simulink model "ammclib_amclib_FW_speed_loop_s32k14x"  (Simulink 9.0)
settings: Solver=FixedStepDiscrete  StartTime=0.0  StopTime=10  FixedStep=0.001  RelTol=1e-3  EnableMultiTasking=on
InitFcn:
  | mbd_s32k_consistency_checks(bdroot(gcs));
undefined symbols (not defined in the file or in its folder): LQFP
libraries: ammclib_bam_s32k14x x8, simulink x4, mbd_s32k1xx_ec_toolbox x2
Description:
  | This model tests the AMMCLIB AMCLIB Field Weakening Speed Loop blocks
  | 
  | Validation:
  | - Run the model in Simulation and compare the Inputs vs Outputs results.
  | - Open Freemaster (ammclib_amclib_FW_speed_loop_s32k14x.pmp) and compare the HW results against the Simulated ones
settings Model: Creator=NXP MBDT Team  LastModifiedBy=nxf35172
settings DataIOCC: ExternalInput=off  InitialState=off  LimitDataPoints=on  SaveOutput=off  SignalLogging=off  SaveTime=off
settings OptimizationCC: DefaultParameterBehavior=Inlined  LifeSpan=1
settings DebuggingCC: SolverPrmCheckMsg=warning  InheritedTsInSrcMsg=none  SingleTaskRateTransMsg=error  ParameterPrecisionLossMsg=none  UnconnectedInputMsg=error  UnconnectedOutputMsg=error  UnconnectedLineMsg=error  AllowSymbolicDim=off  UnknownTsInhSupMsg=error  StateNameClashWarn=warning
settings HardwareCC: ProdLargestAtomicInteger=Long  ProdLargestAtomicFloat=Double  ProdEndianess=LittleEndian  ProdHWDeviceType=ARM Compatible->ARM Cortex
settings SFSimCC: MATLABDynamicMemAlloc=off
settings RTWCC: SystemTargetFile=mbd_s32k.tlc  MakeCommand=mbd_s32k_make_rtw COPY_MDLREF_INCLUDES=0  TemplateMakefile=mbd_s32k.tmf  Description=Model Based Design Toolbox S32K14x Code Generation Target
settings CodeAppCC: IgnoreCustomStorageClasses=off
settings STFCustomTargetCC: CombineOutputUpdateFcns=on  ERTCustomFileBanners=on  SupportContinuousTime=off  SupportNonInlinedSFcns=off  RemoveResetFunc=on  MATLABClassNameForMDSCustomization=Simulink.SoftwareTarget.ERTCustomization  GRTInterface=off  SystemTargetFile=mbd_s32k14.tlc
settings ERTTargetCC: MultiwordLength=2048  ParMdlRefBuildCompliant=off  CompOptLevelCompliant=off  ConcurrentExecutionCompliant=off  ModelStepFunctionPrototypeControlCompliant=off  CPPClassGenCompliant=off  UseToolchainInfoCompliant=off  InlinedParameterPlacement=NonHierarchical  ERTCustomFileTemplate=example_file_process.tlc  ConvertIfToSwitch=off  SuppressUnreachableDefaultCases=off

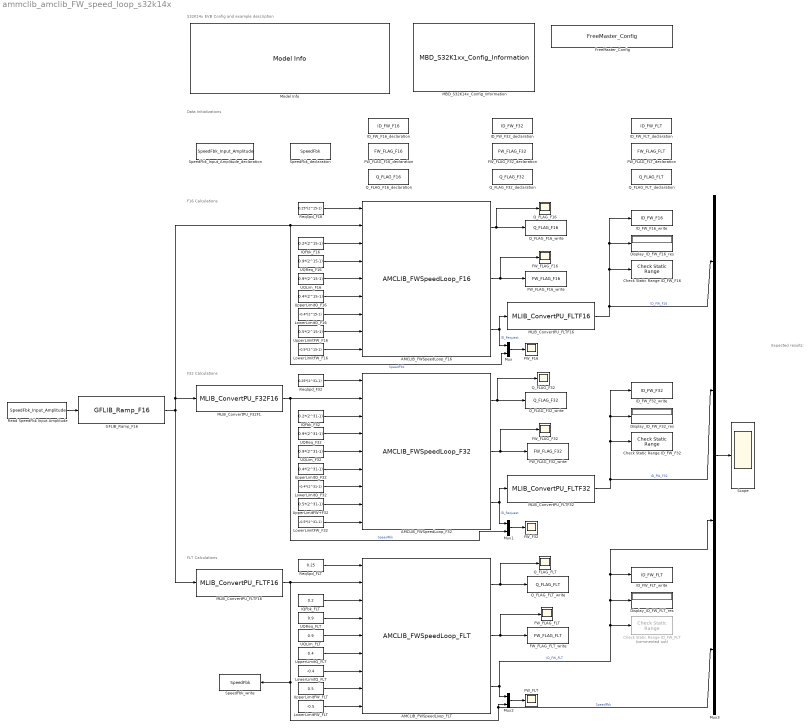
== system ammclib_amclib_FW_speed_loop_s32k14x ==
  note: Expected results:
  note: S32K14x EVB Config and example description
  note: Data Initializations
  note: F16 Calculations
  note: F32 Calculations
  note: FLT Calculations
  AMCLIB_FWSpeedLoop_F16 : ammclib_bam_s32k14x/AMCLIB/bam_f16/AMCLIB_FWSpeedLoop_F16  u16NSamplesW=3  u16NSamplesFW=3  f16PropGainQ=0.001*(2^15-1)  s16PropGainShiftQ=0  f16IntegGainQ=0.0005*(2^15-1)  s16IntegGainShiftQ=0  f16PropGainFW=0.02*(2^15-1)  s16PropGainShiftFW=0  f16IntegGainFW=0.002*(2^15-1)  s16IntegGainShiftFW=0  f32RampUp=0.001*(2^15-1)  f32RampDown=0.001*(2^15-1)
  AMCLIB_FWSpeedLoop_F32 : ammclib_bam_s32k14x/AMCLIB/bam_f32/AMCLIB_FWSpeedLoop_F32  u16NSamplesW=3  u16NSamplesFW=3  f32PropGainQ=0.001*(2^31-1)  s16PropGainShiftQ=0  f32IntegGainQ=0.0005*(2^31-1)  s16IntegGainShiftQ=0  f32PropGainFW=0.02*(2^31-1)  s16PropGainShiftFW=0  f32IntegGainFW=0.002*(2^31-1)  s16IntegGainShiftFW=0  f32RampUp=0.001*(2^31-1)  f32RampDown=0.001*(2^31-1)
  AMCLIB_FWSpeedLoop_FLT : ammclib_bam_s32k14x/AMCLIB/bam_flt/AMCLIB_FWSpeedLoop_FLT  fltLambdaW=0.5  fltLambdaFW=0.5  fltPropGainQ=0.001  fltIntegGainQ=0.0005  fltPropGainFW=0.02  fltIntegGainFW=0.002  fltRampUp=0.001  fltRampDown=0.001  fltUmaxDivImax=1
  "Check Static Range ID_FW_F16 " : simulink/Model Verification/Check  Static Range  Description=0 <= u <= 0.707*(2^15-1)  max=0.707*(2^15-1)  max_included=on  min=0  min_included=on  enabled=on  stopWhenAssertionFail=on  export=off  icon=graphic
      settings: SourceProductName=Simulink  SourceProductBaseCode=SL
  "Check Static Range ID_FW_F32 " : simulink/Model Verification/Check  Static Range  Description=0 <= u <= 0.707*(2^31-1)  max=0.707*(2^31-1)  max_included=on  min=0  min_included=on  enabled=on  stopWhenAssertionFail=on  export=off  icon=graphic
      settings: SourceProductName=Simulink  SourceProductBaseCode=SL
  Check Static Range ID_FW_FLT : simulink/Model Verification/Check  Static Range  Description=0 <= u <= 0.707  Commented=on  max=0.707  max_included=on  min=0  min_included=on  enabled=on  stopWhenAssertionFail=on  export=off  icon=graphic
      settings: SourceProductName=Simulink  SourceProductBaseCode=SL
  Display_ID_FW_F16_res : Display
  Display_ID_FW_F32_res : Display
  Display_ID_FW_FLT_res : Display
  FW_F16 : Scope
  FW_F32 : Scope
  FW_FLAG_F16 : Scope
  FW_FLAG_F16_declaration : DataStoreMemory  Priority=3  DataStoreName=FW_FLAG_F16  ReadBeforeWriteMsg=warning  WriteAfterWriteMsg=warning  WriteAfterReadMsg=warning  ShowAdditionalParam=off  OutDataTypeStr=uint16
  FW_FLAG_F16_write : DataStoreWrite  DataStoreName=FW_FLAG_F16
  FW_FLAG_F32 : Scope
  FW_FLAG_F32_declaration : DataStoreMemory  Priority=3  DataStoreName=FW_FLAG_F32  ReadBeforeWriteMsg=warning  WriteAfterWriteMsg=warning  WriteAfterReadMsg=warning  ShowAdditionalParam=off  OutDataTypeStr=uint16
  FW_FLAG_F32_write : DataStoreWrite  DataStoreName=FW_FLAG_F32
  FW_FLAG_FLT : Scope
  FW_FLAG_FLT_declaration : DataStoreMemory  Priority=3  DataStoreName=FW_FLAG_FLT  ReadBeforeWriteMsg=warning  WriteAfterWriteMsg=warning  WriteAfterReadMsg=warning  ShowAdditionalParam=off  OutDataTypeStr=uint16
  FW_FLAG_FLT_write : DataStoreWrite  DataStoreName=FW_FLAG_FLT
  FW_FLT : Scope
  FreeMaster_Config : mbd_s32k1xx_ec_toolbox/Utility Blocks/FreeMaster_Config  interface=LPUART1  baudrate=115200  rxd=PTC6: [LPUART1_RX | Receive]  txd=PTC7: [LPUART1_TX | Transmit]  mode=Short Interrupt  isr_prio=1  show_adv_opts=on  use_scope=on  max_scope_vars=8  use_recorder=on  max_rec_vars=8  rec_buff_size=1024  rec_timebase=0 milliseconds  comm_buffer_size_auto=on  comm_buffer_size=255  comm_rqueue_size_default=on  comm_rqueue_size=32
  GFLIB_Ramp_F16 : ammclib_bam_s32k14x/GFLIB/bam_f16/GFLIB_Ramp_F16  f16RampUp=2  f16RampDown=2
  ID_FW_F16_declaration : DataStoreMemory  Priority=2  DataStoreName=ID_FW_F16  ReadBeforeWriteMsg=warning  WriteAfterWriteMsg=warning  WriteAfterReadMsg=warning  ShowAdditionalParam=off  OutDataTypeStr=single
  ID_FW_F16_write : DataStoreWrite  DataStoreName=ID_FW_F16
  ID_FW_F32_declaration : DataStoreMemory  Priority=2  DataStoreName=ID_FW_F32  ReadBeforeWriteMsg=warning  WriteAfterWriteMsg=warning  WriteAfterReadMsg=warning  ShowAdditionalParam=off  OutDataTypeStr=single
  ID_FW_F32_write : DataStoreWrite  DataStoreName=ID_FW_F32
  ID_FW_FLT_declaration : DataStoreMemory  Priority=2  DataStoreName=ID_FW_FLT  ReadBeforeWriteMsg=warning  WriteAfterWriteMsg=warning  WriteAfterReadMsg=warning  ShowAdditionalParam=off  OutDataTypeStr=single
  ID_FW_FLT_write : DataStoreWrite  DataStoreName=ID_FW_FLT
  IQFbk_F16 : Constant  Value=0.2*(2^15-1)  OutDataTypeStr=Inherit: Inherit via back propagation
  IQFbk_F32 : Constant  Value=0.2*(2^31-1)  OutDataTypeStr=Inherit: Inherit via back propagation
  IQFbk_FLT : Constant  Value=0.2  OutDataTypeStr=Inherit: Inherit via back propagation
  LowerLimitFW_F16 : Constant  Value=-0.5*(2^15-1)  OutDataTypeStr=Inherit: Inherit via back propagation
  "LowerLimitFW_F32 " : Constant  Value=-0.5*(2^31-1)  OutDataTypeStr=Inherit: Inherit via back propagation
  "LowerLimitFW_FLT  " : Constant  Value=-0.5  OutDataTypeStr=Inherit: Inherit via back propagation
  LowerLimitQ_F16 : Constant  Value=-0.4*(2^15-1)  OutDataTypeStr=Inherit: Inherit via back propagation
  LowerLimitQ_F32 : Constant  Value=-0.4*(2^31-1)  OutDataTypeStr=Inherit: Inherit via back propagation
  LowerLimitQ_FLT : Constant  Value=-0.4  OutDataTypeStr=Inherit: Inherit via back propagation
  MBD_S32K14x_Config_Information : mbd_s32k1xx_ec_toolbox/MBD_S32K1xx_Config_Information  Priority=0  mbdt_ver=0  disp_str=|  config_params=[]  mcu_target_name=S32K144  mcu_target_package=100-LQFP  mcu_target_sram_size=64KB  mcu_system_clock_freq=80  mcu_xtal_freq=External 8  mcu_steptick_timer=LPIT Channel 0  mcu_steptick_prio=15  ds_import_enable=on  target_compiler=GCC  target_memory=FLASH  gcc_target_compile_opts=-mcpu=cortex-m4 -mthumb -mfloat-abi=hard -mfpu=fpv4-sp-d16 -O1 -g -gstrict-dwarf  gcc_target_assemble_opts=-mcpu=cortex-m4 -mthumb -mfloat-abi=hard -mfpu=fpv4-sp-d16 -g  gcc_target_link_opts=-mcpu=cortex-m4 -mthumb -mfloat-abi=hard -mfpu=fpv4-sp-d16  gcc_target_default_lcf=on  gcc_target_user_lcf=S32K144_64_flash.ld  ghs_target_compile_opts=-cpu=cortexm4f -thumb -DARM_MATH_CM4 -fpu=vfpv4_d16 -fsingle -Ogeneral -Wundef -Wimplicit-int -Wshadow -Wtrigraphs --no_commons --gnu_asm -gnu99 -gdwarf-2 -G  ghs_target_assemble_opts=-cpu=cortexm4f -fpu=vfpv4_d16  ghs_target_link_opts=-cpu=cortexm4f -thumb -fpu=vfpv4_d16  ghs_target_default_lcf=off  ghs_target_user_lcf=S32K144_64_flash.ld  iar_target_compile_opts=--cpu=Cortex-M4F --thumb --fpu=VFPv4_sp -Ol -e --debug --dlib_config normal  iar_target_assemble_opts=--cpu Cortex-M4F --thumb --fpu VFPv4_sp  iar_target_link_opts=--no_exceptions --vfe --inline  iar_target_default_lcf=off  iar_target_user_lcf=S32K144_64_flash.icf  pil_download_enable=off  rbl_download_enable=on  rbl_start_delay=5000000  rbl_download_interface=OpenSDA  rbl_restart_request=off  rbl_com_port=Custom  rbl_com_port_custom=COM1  pil_download_rate=57600  pil_opensda_drive=Custom  pil_opensda_drive_custom=D  pil_uart_instance=0  pil_uart_rx=PTA2: [LPUART0_RX | Receive]  pil_uart_tx=PTA3: [LPUART0_TX | Transmit]  FTM_PWM_PcrCheckEnDis=on  FTM_Input_Edge_Inputs_PcrCheckEnDis=on  FTM_Dual_Edge_Inputs_PcrCheckEnDis=on  FTM_Quadrature_Inputs_PcrCheckEnDis=on  FTM_Hall_Sensor_Inputs_PcrCheckEnDis=on  LPTMR_PcrCheckEnDis=on  PIT_PcrCheckEnDis=on  RTC_PcrCheckEnDis=on  FlexCAN_PcrCheckEnDis=on  LIN_PcrCheckEnDis=on  FlexIO_PcrCheckEnDis=on  LPI2C_PcrCheckEnDis=on  LPSPI_PcrCheckEnDis=on  LPUART_PcrCheckEnDis=on  CMP_PcrCheckEnDis=on  GPIO_OutputPcrCheckEnDis=on  GPIO_InputPcrCheckEnDis=on  SBC_PcrCheckEnDis=on  AMMCLIB_PcrCheckEnDis=on  FM_PcrCheckEnDis=on  Profile_PcrCheckEnDis=on  ConfigParams_PcrCheckEnDis=on  ModelRef_PcrCheckEnDis=on  PDB0_PcrCheckEnDis=on  CSEc_PcrCheckEnDis=on  eDMA_PcrCheckEnDis=on  ADC_PcrCheckEnDis=on  WDOG_PcrCheckEnDis=on
      | Target : S32K142-16KB_SRAM
      | Package : 100-pin
      | System clock : 80 MHz
      | XTAL clock : External 8 MHz
      | Compiler : GCC
      | Target Type : FLASH
      | Download Code after build : (OpenSDA: E)
      | Step Tick Interrupt Priority : 15
  MLIB_ConvertPU_F32F1 : ammclib_bam_s32k14x/MLIB/bam_f32/MLIB_ConvertPU_F32F16
  MLIB_ConvertPU_FLTF16 : ammclib_bam_s32k14x/MLIB/bam_flt/MLIB_ConvertPU_FLTF16
  "MLIB_ConvertPU_FLTF16   " : ammclib_bam_s32k14x/MLIB/bam_flt/MLIB_ConvertPU_FLTF16
  MLIB_ConvertPU_FLTF32 : ammclib_bam_s32k14x/MLIB/bam_flt/MLIB_ConvertPU_FLTF32
  Model Info : simulink/Model-Wide Utilities/Model Info  Frame=off  DisplayStringWithTags=|  HorizontalTextAlignment=Left  LeftAlignmentValue=0.02
      | Model Name: %<ModelName>
      | 
      | Description: %<Description>
  Mux : Mux  Inputs=2
  Mux1 : Mux  Inputs=2
  Mux2 : Mux  Inputs=2
  Mux3 : Mux
  Q_FLAG_F16 : Scope
  Q_FLAG_F16_declaration : DataStoreMemory  Priority=3  DataStoreName=Q_FLAG_F16  ReadBeforeWriteMsg=warning  WriteAfterWriteMsg=warning  WriteAfterReadMsg=warning  ShowAdditionalParam=off  OutDataTypeStr=uint16
  Q_FLAG_F16_write : DataStoreWrite  DataStoreName=Q_FLAG_F16
  Q_FLAG_F32 : Scope
  Q_FLAG_F32_declaration : DataStoreMemory  Priority=3  DataStoreName=Q_FLAG_F32  ReadBeforeWriteMsg=warning  WriteAfterWriteMsg=warning  WriteAfterReadMsg=warning  ShowAdditionalParam=off  OutDataTypeStr=uint16
  Q_FLAG_F32_write : DataStoreWrite  DataStoreName=Q_FLAG_F32
  Q_FLAG_FLT : Scope
  Q_FLAG_FLT_declaration : DataStoreMemory  Priority=3  DataStoreName=Q_FLAG_FLT  ReadBeforeWriteMsg=warning  WriteAfterWriteMsg=warning  WriteAfterReadMsg=warning  ShowAdditionalParam=off  OutDataTypeStr=uint16
  Q_FLAG_FLT_write : DataStoreWrite  DataStoreName=Q_FLAG_FLT
  Read SpeedFbk Input Amplitude : DataStoreRead  DataStoreName=SpeedFbk_Input_Amplitude
  ReqSpd_F16 : Constant  Value=0.25*(2^15-1)  OutDataTypeStr=Inherit: Inherit via back propagation
  ReqSpd_F32 : Constant  Value=0.25*(2^31-1)  OutDataTypeStr=Inherit: Inherit via back propagation
  ReqSpd_FLT : Constant  Value=0.25  OutDataTypeStr=Inherit: Inherit via back propagation
  Scope : Scope
  SpeedFbk_Input_Amplitude_declaration : DataStoreMemory  Priority=1  DataStoreName=SpeedFbk_Input_Amplitude  WriteAfterWriteMsg=warning  WriteAfterReadMsg=warning  InitialValue=0.25*(2^15-1)  ShowAdditionalParam=off  OutMin=-32768  OutMax=32767  OutDataTypeStr=int16
  SpeedFbk_declaration : DataStoreMemory  Priority=1  DataStoreName=SpeedFbk  WriteAfterWriteMsg=warning  WriteAfterReadMsg=warning  ShowAdditionalParam=off  OutMin=-1  OutMax=1  OutDataTypeStr=single
  SpeedFbk_write : DataStoreWrite  DataStoreName=SpeedFbk
  UQLim_F16 : Constant  Value=0.9*(2^15-1)  OutDataTypeStr=Inherit: Inherit via back propagation
  UQLim_F32 : Constant  Value=0.9*(2^31-1)  OutDataTypeStr=Inherit: Inherit via back propagation
  UQLim_FLT : Constant  Value=0.9  OutDataTypeStr=Inherit: Inherit via back propagation
  UQReq_F16 : Constant  Value=0.9*(2^15-1)  OutDataTypeStr=Inherit: Inherit via back propagation
  UQReq_F32 : Constant  Value=0.9*(2^31-1)  OutDataTypeStr=Inherit: Inherit via back propagation
  UQReq_FLT : Constant  Value=0.9  OutDataTypeStr=Inherit: Inherit via back propagation
  "UpperLimitFW+F32 " : Constant  Value=0.5*(2^31-1)  OutDataTypeStr=Inherit: Inherit via back propagation
  UpperLimitFW_F16 : Constant  Value=0.5*(2^15-1)  OutDataTypeStr=Inherit: Inherit via back propagation
  "UpperLimitFW_FLT   " : Constant  Value=0.5  OutDataTypeStr=Inherit: Inherit via back propagation
  UpperLimitQ_F16 : Constant  Value=0.4*(2^15-1)  OutDataTypeStr=Inherit: Inherit via back propagation
  UpperLimitQ_F32 : Constant  Value=0.4*(2^31-1)  OutDataTypeStr=Inherit: Inherit via back propagation
  UpperLimitQ_FLT : Constant  Value=0.4  OutDataTypeStr=Inherit: Inherit via back propagation
  wires:
  UpperLimitFW_F16/1 -> AMCLIB_FWSpeedLoop_F16/8
  LowerLimitFW_F16/1 -> AMCLIB_FWSpeedLoop_F16/9
  AMCLIB_FWSpeedLoop_F16/2 -> FW_FLAG_F16/1, FW_FLAG_F16_write/1
  Read SpeedFbk Input Amplitude/1 -> GFLIB_Ramp_F16/1
  ReqSpd_F16/1 -> AMCLIB_FWSpeedLoop_F16/1
  AMCLIB_FWSpeedLoop_F16/3 -> "MLIB_ConvertPU_FLTF16   "/1, Mux/1  "ID_Request"
  "MLIB_ConvertPU_FLTF16   "/1 -> "Check Static Range ID_FW_F16 "/1, Display_ID_FW_F16_res/1, ID_FW_F16_write/1, Mux3/1  "ID_FW_F16"
  Mux/1 -> FW_F16/1
  Mux3/1 -> Scope/1
  GFLIB_Ramp_F16/1 -> Mux/2, AMCLIB_FWSpeedLoop_F16/2, MLIB_ConvertPU_F32F1/1, MLIB_ConvertPU_FLTF16/1  "SpeedFbk"
  IQFbk_F16/1 -> AMCLIB_FWSpeedLoop_F16/3
  UQLim_F16/1 -> AMCLIB_FWSpeedLoop_F16/5
  UQReq_F16/1 -> AMCLIB_FWSpeedLoop_F16/4
  "UpperLimitFW+F32 "/1 -> AMCLIB_FWSpeedLoop_F32/8
  "LowerLimitFW_F32 "/1 -> AMCLIB_FWSpeedLoop_F32/9
  AMCLIB_FWSpeedLoop_F32/2 -> FW_FLAG_F32/1, FW_FLAG_F32_write/1
  ReqSpd_F32/1 -> AMCLIB_FWSpeedLoop_F32/1
  AMCLIB_FWSpeedLoop_F32/3 -> MLIB_ConvertPU_FLTF32/1, Mux1/1  "ID_Request"
  MLIB_ConvertPU_FLTF32/1 -> Display_ID_FW_F32_res/1, ID_FW_F32_write/1, "Check Static Range ID_FW_F32 "/1, Mux3/2  "ID_FW_F32"
  Mux1/1 -> FW_F32/1
  MLIB_ConvertPU_F32F1/1 -> Mux1/2, AMCLIB_FWSpeedLoop_F32/2  "SpeedFbk"
  IQFbk_F32/1 -> AMCLIB_FWSpeedLoop_F32/3
  UQLim_F32/1 -> AMCLIB_FWSpeedLoop_F32/5
  UQReq_F32/1 -> AMCLIB_FWSpeedLoop_F32/4
  "UpperLimitFW_FLT   "/1 -> AMCLIB_FWSpeedLoop_FLT/8
  "LowerLimitFW_FLT  "/1 -> AMCLIB_FWSpeedLoop_FLT/9
  AMCLIB_FWSpeedLoop_FLT/2 -> FW_FLAG_FLT/1, FW_FLAG_FLT_write/1
  ReqSpd_FLT/1 -> AMCLIB_FWSpeedLoop_FLT/1
  AMCLIB_FWSpeedLoop_FLT/3 -> Mux3/3, ID_FW_FLT_write/1, Display_ID_FW_FLT_res/1, Check Static Range ID_FW_FLT/1, Mux2/1  "ID_FW_FLT"
  Mux2/1 -> FW_FLT/1
  MLIB_ConvertPU_FLTF16/1 -> SpeedFbk_write/1, Mux2/2, Mux3/4, AMCLIB_FWSpeedLoop_FLT/2  "SpeedFbk"
  IQFbk_FLT/1 -> AMCLIB_FWSpeedLoop_FLT/3
  UQLim_FLT/1 -> AMCLIB_FWSpeedLoop_FLT/5
  UQReq_FLT/1 -> AMCLIB_FWSpeedLoop_FLT/4
  UpperLimitQ_F16/1 -> AMCLIB_FWSpeedLoop_F16/6
  LowerLimitQ_F16/1 -> AMCLIB_FWSpeedLoop_F16/7
  AMCLIB_FWSpeedLoop_F16/1 -> Q_FLAG_F16/1, Q_FLAG_F16_write/1
  AMCLIB_FWSpeedLoop_F32/1 -> Q_FLAG_F32/1, Q_FLAG_F32_write/1
  UpperLimitQ_F32/1 -> AMCLIB_FWSpeedLoop_F32/6
  LowerLimitQ_F32/1 -> AMCLIB_FWSpeedLoop_F32/7
  AMCLIB_FWSpeedLoop_FLT/1 -> Q_FLAG_FLT/1, Q_FLAG_FLT_write/1
  UpperLimitQ_FLT/1 -> AMCLIB_FWSpeedLoop_FLT/6
  LowerLimitQ_FLT/1 -> AMCLIB_FWSpeedLoop_FLT/7
